simulink subsystem "hexa_prop_forces_moments"  (R2024a)
settings: Solver=VariableStepAuto  StartTime=0.0  StopTime=10.0  RelTol=1e-3
values from neighbouring files (symbols this model uses):
  armLength = 0.275    [F550_data.m]
  motorJm = 0.0001287    [F550_data.m]
settings Model: Creator=user  LastModifiedBy=user

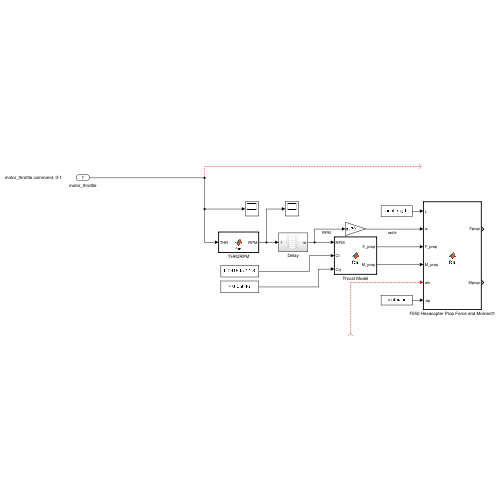
[thumbnail: Simulink's stored preview of the top-level diagram]
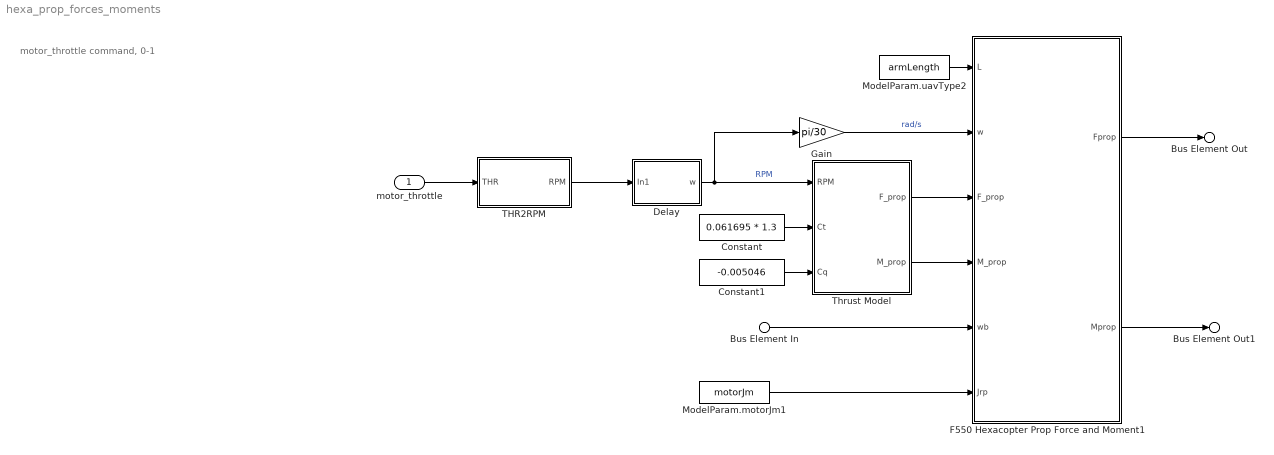
== system hexa_prop_forces_moments ==
  note: motor_throttle command, 0-1
  motor_throttle : Inport  PortDimensions=[1 6]
  Bus Element In : Inport  Port=2  PortName=States  Element=PQR
  Constant : Constant  Value=0.061695 * 1.3
  Constant1 : Constant  Value=-0.005046
  Delay : Subsystem
  F550 Hexacopter Prop Force and Moment1 : MATLAB Function  TreatAsAtomicUnit=on
  Gain : Gain  Gain=pi/30
  ModelParam.motorJm1 : Constant  Value=motorJm
  ModelParam.uavType2 : Constant  Value=armLength
  THR2RPM : MATLAB Function  TreatAsAtomicUnit=on
  Thrust Model : MATLAB Function  TreatAsAtomicUnit=on
  Bus Element Out : Outport  PortName=FM_prop  Element=F_xyz
  Bus Element Out1 : Outport  PortName=FM_prop  Element=M_xyz
  wires:
  Gain/1 -> F550 Hexacopter Prop Force and Moment1/2(w)  "rad/s"
  Delay/1(w) -> Thrust Model/1(RPM), Gain/1  "RPM"
  THR2RPM/1(RPM) -> Delay/1(In1)
  Constant1/1 -> Thrust Model/3(Cq)
  ModelParam.motorJm1/1 -> F550 Hexacopter Prop Force and Moment1/6(Jrp)
  ModelParam.uavType2/1 -> F550 Hexacopter Prop Force and Moment1/1(L)
  Thrust Model/2(M_prop) -> F550 Hexacopter Prop Force and Moment1/4(M_prop)
  motor_throttle/1 -> THR2RPM/1(THR)
  Thrust Model/1(F_prop) -> F550 Hexacopter Prop Force and Moment1/3(F_prop)
  Constant/1 -> Thrust Model/2(Ct)
  Bus Element In/1 -> F550 Hexacopter Prop Force and Moment1/5(wb)
  F550 Hexacopter Prop Force and Moment1/1(Fprop) -> Bus Element Out/1
  F550 Hexacopter Prop Force and Moment1/2(Mprop) -> Bus Element Out1/1

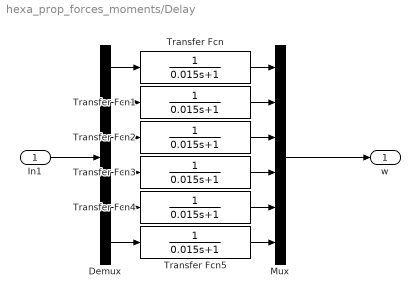
== system hexa_prop_forces_moments/Delay ==
  In1 : Inport
  Demux : Demux  Outputs=6
  Mux : Mux  Inputs=6
  Transfer Fcn{,1..5} (6 alike) : TransferFcn  Denominator=[0.015 1]
  w : Outport
  wires:
  In1/1 -> Demux/1
  Mux/1 -> w/1
  Transfer Fcn/1 -> Mux/1
  Demux/1 -> Transfer Fcn/1
  Demux/2 -> Transfer Fcn1/1
  Demux/3 -> Transfer Fcn2/1
  Demux/4 -> Transfer Fcn3/1
  Demux/5 -> Transfer Fcn4/1
  Demux/6 -> Transfer Fcn5/1
  Transfer Fcn1/1 -> Mux/2
  Transfer Fcn2/1 -> Mux/3
  Transfer Fcn3/1 -> Mux/4
  Transfer Fcn4/1 -> Mux/5
  Transfer Fcn5/1 -> Mux/6

== matlab function hexa_prop_forces_moments/F550 Hexacopter Prop Force and Moment1 ==
  data: L input; w input; F_prop input; M_prop input; Fprop output; Mprop output; wb input; Jrp input
function [Fprop, Mprop] = fcn(L, w, F_prop, M_prop, wb, Jrp)

 % Body Frame : NED Coordinate
 % X-axis : Heading, Y-axis : Right wing, Z-axis : Down

 %  Obtain the force and torque acting on the body. 
 %  The airframe of the hexarotor is as follows: PX4 Hexacopter Configuration
 %     3↓   5↑
 %      \  /
 %   2↑--  -- 1↓
 %      /  \
 %     6↓   4↑
 %  ↑ stands for counterclockwise and ↓stands for clockwise.


 % Input：
 %  w: motor speed，unit：rad/s
 %  L: Arm Length (m) - In case of F550 R = 0.275 m
 %  Cm: torque coefficient
 %  Ct: thrust coefficient
 %  wb: angular velocity in the body coordinate system
 %  Jrp:  moment of inertia of motor rotor + propeller

 % Output:
 %  Fprop: force vector from prop [6x1] vector
 %  Mprop: aerodynamic damping moment + gyro moment
        
        % Legacy Code - From F450 Quadcopter 
        %  F_prop = Ct*(w.^2);      % Force from each prop
        %  M_prop = Cm*(w.^2);      % Torque magnitude from each prop
        % 
        %  Fprop = [0; 0; -sum(F_prop)];
        % 
        %  d=sin(pi/4)*R;
        %  Mp= [ d*F_prop'*[-1;  1;  1; -1]
        %        d*F_prop'*[ 1; -1;  1; -1]
        %          M_prop'*[ 1;  1; -1; -1] ];
        % 
        % % gyro moment
        %  M_gyro   = [Jrp*wb(2)*( w(1) + w(2) - w(3) - w(4));  
        %              Jrp*wb(1)*(-w(1) - w(2) + w(3) + w(4));
        %              0];
        % 
        %  Mprop = Mp + M_gyro;

    % 프로펠러에 의한 힘 
    Fprop = [0; 0; -sum(F_prop)];
    
    % 로터에 추력/회전에 의해 기체에 작용하는 모멘트
    Mp = [ F_prop'*[-L; L; 0.5*L; -0.5*L; -0.5*L; 0.5*L]
           F_prop'*[0; 0; sqrt(3)/2*L; -sqrt(3)/2*L; sqrt(3)/2*L; -sqrt(3)/2*L]
           M_prop'*[-1; 1; -1; 1; 1; -1;]
         ];
    
    % 동체 회전에 의해 회전하는 프롭에 작용하는 모멘트
    M_gyro = [Jrp*wb(2)*( -w(1)+w(2)-w(3)+w(4)+w(5)-w(6) );
              -Jrp*wb(1)*( -w(1)+w(2)-w(3)+w(4)+w(5)-w(6));
              0;
        ];
    
    Mprop = Mp + M_gyro;
end

== matlab function hexa_prop_forces_moments/THR2RPM ==
  data: THR input; RPM output
function RPM = fcn(THR)
u = 1000*THR + 1000;

RPM = -0.0028021742*u.^2 + 15.0583283059*u - 10837.5342615064;

== matlab function hexa_prop_forces_moments/Thrust Model ==
  data: RPM input; F_prop output; Ct input; Cq input; M_prop output
function [F_prop, M_prop] = fcn(RPM, Ct, Cq)
inch2m = 0.0254;

n = RPM ./ 60;
rho = 1.225;
D = 10 * inch2m;

F_prop = Ct * rho * D^4 * n.^2;

M_prop = -Cq * rho * D^5 * n.^2;
